simulink model "power_SwitchedReluctanceMotor"  (R2020a)
settings: Solver=FixedStepAuto  StartTime=0.0  StopTime=1  FixedStep=Ts  RelTol=1e-3  AbsTol=1e-5  EnableMultiTasking=on
PreLoadFcn:
  | Ts=1e-6;
  | 
  | % Magnetisation characteristic table of the switched Reluctance Motor:
  | % Table elements =  Flux linkage, in Wb.
  | 
  | FTBL = [
  |     0             0              0             0             0             0
  |     0.3220    0.3050    0.2280    0.1240    0.0220    0.0170
  |     0.3760    0.3570    0.2770    0.1600    0.0420    0.0340
  |     0.3990    0.3850    0.3000    0.1830    0.0640    0.0500
  |     0.4160    0.4020    0.3200    0.2010    0.0840    0.0670
  |     0.4280    0.4150    0.3340    0.2190    0.1030    0.0840
  |     0.4370    0.4260    0.3480    0.2370    0.1230    0.1010
  |     0.4430    0.4330    0.3590    0.2530    0.1420    0.1170
  |     0.4490    0.4390    0.3710    0.2680    0.1610    0.1340
  |     0.4540    0.4440    0.3820    0.2820    0.1790    0.1510
  |     0.4590    0.4490    0.3920    0.2950    0.1970    0.1680
  |     0.4630    0.4530    0.4020    0.3090    0.2140    0.1840
  |     0.4670    0.4570    0.4110    0.3220    0.2310    0.2010
  |     0.4700    0.4620    0.4190    0.3360    0.2460    0.2180
  |     0.4740    0.4650    0.4270    0.3480    0.2610    0.2350
  |     0.4780    0.4690    0.4330    0.3590    0.2770    0.2510
  |     0.4810    0.4730    0.4380    0.3690    0.2910    0.2680
  |     0.4840    0.4770    0.4440    0.3800    0.3050    0.2850
  |     0.4870    0.4790    0.4480    0.3890    0.3200    0.3020];
  | 
  | % Table columns :  Rotor angles, in degrees.
  | 
  | RotorAngles = [
  |     0             10            20            30            40            45];
  | 
  | % Table rows : Stator current, in A.
  | 
  | StatorCurrents = [ 0:size(FTBL,1)-1] * 25;
  | 
  | % In the Switched Reluctance Motor block, select the "plot magnetization curves"
  | % to plot the corresponding characteristic of the above table.
undefined symbols (not defined in the file): DiscIntNeverNeededParam, find_system
libraries: powerlib x40, simulink x3, powerlib_meascontrol x1
settings Model: ExtModeAutoUpdateStatusClock=off  Creator=MathWorks  LastModifiedBy=mahfo
settings SolverCC: AutoScaleAbsTol=off  InsertRTBMode=Auto
settings DataIOCC: LimitDataPoints=on  SaveFormat=Array  SignalLoggingSaveFormat=ModelDataLogs  ReturnWorkspaceOutputs=off  SignalLoggingName=sigsOut
settings OptimizationCC: ExpressionDepthLimit=2147483647  InitFltsAndDblsToZero=on  LifeSpan=inf
settings DebuggingCC: UnderspecifiedInitializationDetection=Classic  MergeDetectMultiDrivingBlocksExec=none  CheckExecutionContextPreStartOutputMsg=on  CheckExecutionContextRuntimeOutputMsg=on  SignalResolutionControl=TryResolveAllWithWarning  MultiTaskDSMMsg=warning  MultiTaskCondExecSysMsg=none  FcnCallInpInsideContextMsg=warning  StateNameClashWarn=warning  SFUnexpectedBacktrackingDiag=warning  SFNoUnconditionalDefaultTransitionDiag=warning  SFExecutionAtInitializationDiag=none  ArithmeticOperatorsInVariantConditions=warning
settings HardwareCC: ProdBitPerPointer=32  ProdBitPerSizeT=32  ProdBitPerPtrDiffT=32  ProdLargestAtomicFloat=None  ProdIntDivRoundTo=Undefined  ProdEndianess=Unspecified  ProdWordSize=32  ProdHWDeviceType=32-bit Generic  TargetUnknown=on
settings ModelReferenceCC: PropagateSignalLabelsOutOfModel=off
settings SFSimCC: SimUseLocalCustomCode=off  CustomCodeUndefinedFunction=UseInterfaceOnly
settings RTWCC: RTWUseLocalCustomCode=off
settings CodeAppCC: StateflowObjectComments=on
settings GRTTargetCC: TargetLangStandard=C89/C90 (ANSI)  CombineOutputUpdateFcns=off  GRTInterface=on
settings ConfigComp: CovMetricSettings=dw  CovHtmlReporting=on  CovSaveCumulativeToWorkspaceVar=on  CovSaveSingleToWorkspaceVar=on  CovExternalEMLEnable=off  CovSFcnEnable=off
settings SimscapeCC: SimscapeNormalizeSystem=off

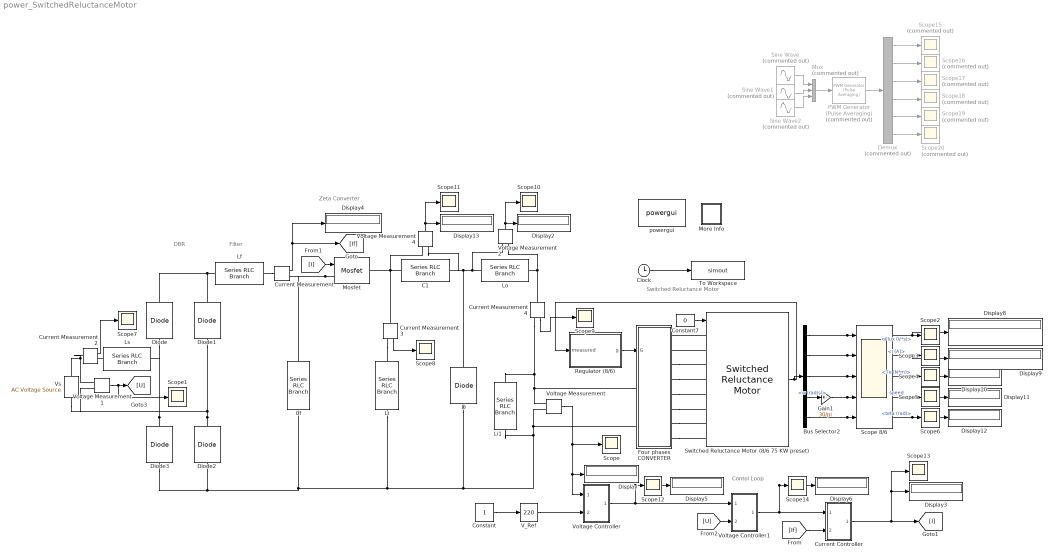
== system power_SwitchedReluctanceMotor ==
  note: Switched Reluctance Motor
  note: Filter
  note: Zeta Converter
  note: DBR
  note: Contol Loop
  Bus Selector2 : BusSelector  OutputSignals=Flux (V*s),I (A),Te (N*m),w (rad/s),teta (rad)
  C1 : powerlib/Elements/Series RLC Branch  LConnTagsString=__new0  RConnTagsString=__new0  BranchType=C  Resistance=1  Inductance=1e-3  SetiL0=off  InitialCurrent=0  Capacitance=1.48e-6  Setx0=off  InitialVoltage=0  Measurements=None
  Cf : powerlib/Elements/Series RLC Branch  LConnTagsString=__new0  RConnTagsString=__new0  BranchType=C  Resistance=1  Inductance=1e-3  SetiL0=off  InitialCurrent=0  Capacitance=1e-6  Setx0=off  InitialVoltage=0  Measurements=None
  Clock : Clock
  Constant : Constant
  Constant7 : Constant  Value=0
  Current Controller : Subsystem
  Current Measurement{,2..4} (4 alike) : powerlib/Measurements/Current Measurement  PhasorSimulation=off  OutputType=Complex  PSBequivalent=0
  D : powerlib/Power Electronics/Diode  Ron=0.001  Lon=0  Vf=0.8  IC=0  UseSnubber=0  Rs=500  Cs=250e-9  Measurements=off
  Demux : Demux  Commented=on  Outputs=6
  Diode{,1..3} (4 alike) : powerlib/Power Electronics/Diode  Ron=0.001  Lon=0  Vf=0.8  IC=0  UseSnubber=0  Rs=500  Cs=250e-9  Measurements=off
  Display{,2..6,8..13} (12 alike) : Display
  Four phases CONVERTER : Subsystem  LoadFcn=find_system(gcs,'FollowLinks', 'on', 'LookUnderMasks', 'all');
  Gain1 : Gain  Gain=30/pi  SaturateOnIntegerOverflow=on  OutDataTypeStr=Inherit: Same as input  ParamDataTypeStr=Inherit: Same as input
  Lf : powerlib/Elements/Series RLC Branch  LConnTagsString=__new0  RConnTagsString=__new0  BranchType=L  Resistance=1  Inductance=1.37e-3  SetiL0=off  InitialCurrent=0  Capacitance=1e-6  Setx0=off  InitialVoltage=0  Measurements=None
  Li : powerlib/Elements/Series RLC Branch  LConnTagsString=__new0  RConnTagsString=__new0  BranchType=L  Resistance=1  Inductance=1e-3  SetiL0=off  InitialCurrent=0  Capacitance=1e-6  Setx0=off  InitialVoltage=0  Measurements=None
  Li1 : powerlib/Elements/Series RLC Branch  LConnTagsString=__new0  RConnTagsString=__new0  BranchType=C  Resistance=10  Inductance=100  SetiL0=off  InitialCurrent=0  Capacitance=1500e-6  Setx0=off  InitialVoltage=0  Measurements=None
  Lo : powerlib/Elements/Series RLC Branch  LConnTagsString=__new0  RConnTagsString=__new0  BranchType=L  Resistance=1  Inductance=4.51e-3  SetiL0=off  InitialCurrent=0  Capacitance=1e-6  Setx0=off  InitialVoltage=0  Measurements=None
  Ls : powerlib/Elements/Series RLC Branch  LConnTagsString=__new0  RConnTagsString=__new0  BranchType=L  Resistance=1  Inductance=4.38e-3  SetiL0=off  InitialCurrent=0  Capacitance=1e-6  Setx0=off  InitialVoltage=0  Measurements=None
  More Info : Subsystem
      settings: OpenFcn=showdemo(bdroot(gcb))
      mask Display: disp('?')
  Mosfet : powerlib/Power Electronics/Mosfet  Ron=0.1  Lon=0  Rd=0.01  Vfd=0  IC=0  Rs=1e5  Cs=inf  Measurements=off
  Mux : Mux  Commented=on  Inputs=3
  PWM Generator (Pulse Averaging) : powerlib_meascontrol/Pulse & Signal Generators/PWM Generator (Pulse Averaging)  Commented=on  GeneratorType=Two-level, three-phase  Fc=2000  InitialPhase=0  Ts=Ts
      settings: SourceProductBaseCode=PS
  Regulator (8/6) : Subsystem  mask{Iref=50, initpos=[0,-15,-30,-45], TurnOn=37.5, TurnOff=52.5}
      mask prompts: Iref "Reference current"; initpos "initial positions"; TurnOn "Turn-on angle (deg)"; TurnOff "Turn-off angle (deg)"
  Scope{,1..14} (15 alike) : Scope
  Scope 8/6 : Scope  NumInputPorts=5
  Scope{15..20} (6 alike) : Scope  Commented=on
  Sine Wave : Sin  Commented=on  SampleTime=0
  Sine Wave1 : Sin  Commented=on  SampleTime=0
  Sine Wave2 : Sin  Commented=on  SampleTime=0
  Switched Reluctance Motor (8/6 75 KW preset) : powerlib/Machines/Switched Reluctance Motor  MachineType="8/6  (75 kw preset model)"  StatorResistance=0.05  Inertia=0.01  Friction=0.005  InitialSpeed=[0,0]  TsPowergui=0  TsBlock=Ts  MachineModel=Specific model  Lq=0.67e-3  Ld=23.6e-3  Lsat=0.15e-3  MaximumCurrent=450  MaximumFluxLinkage=0.486  Source=Dialog  MagnetisationCharacteristic=FTBL  RotorAngleVector=RotorAngles  StatorCurrentVector=StatorCurrents  PlotCurves=off
      settings: SourceProductBaseCode=MT,PS
  To Workspace : ToWorkspace  VariableName=simout  SaveFormat=Timeseries  SampleTime=-1
  V_Ref : simulink/Math Operations/Slider Gain  gain=220  low=0  high=440
  Voltage Controller : Subsystem
  Voltage Controller1 : Subsystem
  Voltage Measurement{,1..2,4} (4 alike) : powerlib/Measurements/Voltage Measurement  PhasorSimulation=off  OutputType=Complex  PSBequivalent=0
  Vs : powerlib/Electrical Sources/AC Voltage Source  Amplitude=320  Phase=0  Frequency=200  SampleTime=0  Measurements=None  BusType=swing  Pref=10e3  Qref=0  Qmin=-inf  Qmax=+inf
  powergui : powerlib/powergui  Priority=2  SimulationMode=Discrete  SampleTime=Ts  frequency=60  Iterations=50  frequencyindice=0  Pbase=100e6  ErrMax=1e-4  UnitsV=kV  UnitsW=MW  buscounter=0  FunctionMessages=off  echomessages=off  EnableUseOfTLC=off  CurrentSourceSwitches=off  DisableSnubberDevices=off  DisableRonSwitches=off  DisableVfSwitches=off  DisplayEquations=off  AutomaticDiscreteSolvers=off  SolverType=Tustin/Backward Euler (TBE)  Interpol=off  ExternalGateDelay=off  methode=off  Ts=0  x0status=blocks  SPID=off  SwTol=0  HookPort=off  NonlinearTolerance=0  nMaxIteration=15  ContinueOnMaxIteration=off  RestoreLinks=warning  ResistiveCurrentMeasurement=off  Frange=[0:2:500]  Ylog=off  Xlog=on  ShowGrid=off  save=off  variable=ZData  structure=0  ZoomFFT=on  StartTime=0.0  cycles=1  DisplayStyle=1  fundamental=60  FreqAxis=off  MaxFrequency=1000  frequencyindicesteady=1  RmsSteady=1  display=off
  wires:
  Constant7/1 -> Switched Reluctance Motor (8/6 75 KW preset)/1
  Switched Reluctance Motor (8/6 75 KW preset)/1 -> Bus Selector2/1, Regulator (8/6)/1(measured)
  Regulator (8/6)/1(g) -> Four phases CONVERTER/1(G)
  Bus Selector2/1 -> Display8/1, Scope2/1, Scope 8/6/1  "<Flux (V*s)>"
  Bus Selector2/2 -> Scope 8/6/2, Display9/1, Scope3/1  "<I (A)>"
  Bus Selector2/3 -> Display10/1, Scope4/1, Scope 8/6/3  "<Te (N*m)>"
  Bus Selector2/4 -> Gain1/1  "<w (rad/s)>"
  Gain1/1 -> Display11/1, Scope5/1, Scope 8/6/4  "speed"
  ? -> ?
  Voltage Measurement/1 -> Voltage Controller/1(In1), Display/1, Scope/1
  Bus Selector2/5 -> Scope 8/6/5, Display12/1, Scope6/1  "<teta (rad)>"
  Current Measurement/1 -> Display4/1, [If]
  [If] -> Current Controller/2(In2)
  Current Controller/1(Out1) -> Display3/1, Scope13/1, [I]
  Clock/1 -> To Workspace/1
  Constant/1 -> V_Ref/1
  V_Ref/1 -> Voltage Controller/2(In2)
  Voltage Measurement1/1 -> Scope1/1, [U]
  Voltage Controller/1(Out1) -> Voltage Controller1/1(In1), Display5/1, Scope12/1
  [U] -> Voltage Controller1/2(In2)
  Current Measurement2/1 -> Scope7/1
  Current Measurement3/1 -> Scope8/1
  Current Measurement4/1 -> Scope9/1
  Voltage Measurement2/1 -> Scope10/1, Display2/1
  Voltage Measurement4/1 -> Display13/1, Scope11/1
  PWM Generator (Pulse Averaging)/1 -> Demux/1
  Sine Wave/1 -> Mux/1
  Sine Wave1/1 -> Mux/2
  Sine Wave2/1 -> Mux/3
  Mux/1 -> PWM Generator (Pulse Averaging)/1
  Demux/1 -> Scope15/1
  Demux/2 -> Scope16/1
  Demux/3 -> Scope17/1
  Demux/4 -> Scope18/1
  Demux/5 -> Scope19/1
  Demux/6 -> Scope20/1
  Voltage Controller1/1(Out1) -> Current Controller/1(In1), Display6/1, Scope14/1
  [I] -> Mosfet/1
  connections:
  Switched Reluctance Motor (8/6 75 KW preset)/LConn2 -- Four phases CONVERTER/RConn2
  Four phases CONVERTER/RConn3 -- Switched Reluctance Motor (8/6 75 KW preset)/LConn3
  Switched Reluctance Motor (8/6 75 KW preset)/LConn1 -- Four phases CONVERTER/RConn1
  Four phases CONVERTER/RConn4 -- Switched Reluctance Motor (8/6 75 KW preset)/LConn4
  Four phases CONVERTER/RConn5 -- Switched Reluctance Motor (8/6 75 KW preset)/LConn5
  Four phases CONVERTER/RConn6 -- Switched Reluctance Motor (8/6 75 KW preset)/LConn6
  Four phases CONVERTER/RConn7 -- Switched Reluctance Motor (8/6 75 KW preset)/LConn7
  Four phases CONVERTER/RConn8 -- Switched Reluctance Motor (8/6 75 KW preset)/LConn8
  Current Measurement4/LConn1 -- Voltage Measurement2/LConn2 -- Lo/RConn1
  Mosfet/LConn1 -- Current Measurement/RConn1 -- Cf/LConn1
  C1/LConn1 -- Voltage Measurement4/LConn2 -- Current Measurement3/LConn1 -- Mosfet/RConn1
  Diode2/RConn1 -- Vs/LConn1 -- Voltage Measurement1/LConn2 -- Diode1/LConn1
  Lo/LConn1 -- Voltage Measurement4/LConn1 -- C1/RConn1 -- D/RConn1 -- Voltage Measurement2/LConn1
  Diode/RConn1 -- Lf/LConn1 -- Diode1/RConn1
  Diode3/RConn1 -- Diode/LConn1 -- Ls/RConn1
  Voltage Measurement1/LConn1 -- Current Measurement2/LConn1 -- Vs/RConn1
  Voltage Measurement/LConn2 -- Four phases CONVERTER/LConn2 -- Li1/LConn1 -- D/LConn1 -- Li/LConn1 -- Diode3/LConn1 -- Diode2/LConn1 -- Cf/RConn1
  Current Measurement2/RConn1 -- Ls/LConn1
  Current Measurement4/RConn1 -- Voltage Measurement/LConn1 -- Four phases CONVERTER/LConn1 -- Li1/RConn1
  Current Measurement3/RConn1 -- Li/RConn1
  Lf/RConn1 -- Current Measurement/LConn1

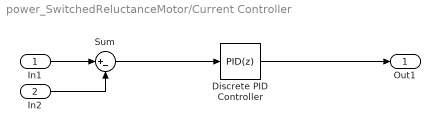
== system power_SwitchedReluctanceMotor/Current Controller ==
  In1 : Inport
  In2 : Inport  Port=2
  Discrete PID Controller : simulink/Continuous/PID Controller  Controller=PID  Form=Parallel  TimeDomain=Discrete-time  UseExternalTs=off  SampleTime=-1  IntegratorMethod=Forward Euler  FilterMethod=Forward Euler  ControllerParametersSource=internal  P=1  I=1  D=0  UseFilter=on  N=100  TunerSelectOption=Transfer Function Based (PID Tuner App)  InitialConditionSource=internal  InitialConditionForIntegrator=0  InitialConditionForFilter=0  DifferentiatorICPrevScaledInput=0  ExternalReset=none  TrackingMode=off  Kt=1  LimitOutput=off  UpperSaturationLimit=inf  LowerSaturationLimit=-inf  LinearizeAsGain=off  AntiWindupMode=none  Kb=1  POutMin=[]  POutMax=[]  IOutMin=[]  IOutMax=[]  DOutMin=[]  DOutMax=[]  NOutMin=[]  NOutMax=[]  SumOutMin=[]  SumOutMax=[]  SaturationOutMin=[]  SaturationOutMax=[]  PParamMin=[]  PParamMax=[]  IParamMin=[]  IParamMax=[]  DParamMin=[]  DParamMax=[]  NParamMin=[]  NParamMax=[]  KbParamMin=[]  KbParamMax=[]  KtParamMin=[]  KtParamMax=[]  KbOutMin=[]  KbOutMax=[]  KtOutMin=[]  KtOutMax=[]  IntegratorOutMin=[]  IntegratorOutMax=[]  FilterOutMin=[]  FilterOutMax=[]  SumI1OutMin=[]  SumI1OutMax=[]  SumI2OutMin=[]  SumI2OutMax=[]  SumI3OutMin=[]  SumI3OutMax=[]  SumI4OutMin=[]  SumI4OutMax=[]  SumDOutMin=[]  SumDOutMax=[]  DifferentiatorOutMin=[]  DifferentiatorOutMax=[]  FilterDiffOutCoefMin=[]  FilterDiffOutCoefMax=[]  ReciprocalOutMin=[]  ReciprocalOutMax=[]  SumDenOutMin=[]  SumDenOutMax=[]  SumNumOutMin=[]  SumNumOutMax=[]  DivideOutMin=[]  DivideOutMax=[]  UdiffTsProdOutMin=[]  UdiffTsProdOutMax=[]  NTsProdOutMin=[]  NTsProdOutMax=[]  UintegralTsProdOutMin=[]  UintegralTsProdOutMax=[]  UngainTsProdOutMin=[]  UngainTsProdOutMax=[]  IntegratorContinuousStateAttributes=''  IntegratorStateMustResolveToSignalObject=off  IntegratorRTWStateStorageClass=Auto  FilterContinuousStateAttributes=''  FilterStateMustResolveToSignalObject=off  FilterRTWStateStorageClass=Auto  ParallelPVariant=InternalParameters  IdealPVariant=Disabled  IVariant=InternalParameters  DVariant=InternalParameters  IntegratorVariant=Discrete  SatVariant=Disabled  AWVariant=Passthrough  PCopyVariant=Disabled  TRVariant=Disabled  FdbkBlocksVariant=Forward  IdealPFdbkVariant=Disabled  SatFdbkVariant=Disabled  DerivativeFilterVariant=ForwardEulerFilter  NVariant=InternalParameters  NCopyVariant=Disabled  FilterICVariant=InternalICsFilter  IntegratorICVariant=InternalICs  ExternalResetVariant=Disabled  TRSumVariant=Passthrough  SumFdbkVariant=Disabled  SumVariant=Sum_PID  TsampFilterVariant=InternalTs  TsampNgainVariant=Passthrough  TsampIntegralVariant=Passthrough
  Sum : Sum  Inputs=|+-
  Out1 : Outport
  wires:
  Sum/1 -> Discrete PID Controller/1
  In1/1 -> Sum/1
  In2/1 -> Sum/2
  Discrete PID Controller/1 -> Out1/1

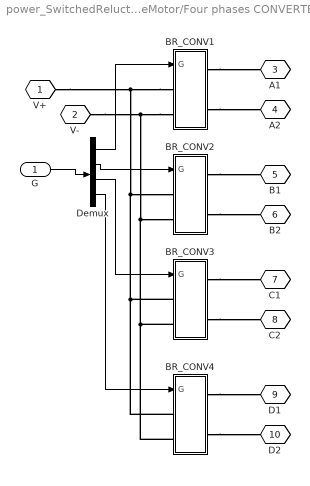
== system power_SwitchedReluctanceMotor/Four phases CONVERTER ==
  G : Inport
  BR_CONV1 : Subsystem
  BR_CONV2 : Subsystem
  BR_CONV3 : Subsystem
  BR_CONV4 : Subsystem
  Demux : Demux
      settings: DisplayOption=none
  V+ : PMIOPort  Tag=PMCPort  Side=Left
  V- : PMIOPort  Tag=PMCPort  Port=2  Side=Left
  A1 : PMIOPort  Tag=PMCPort  Port=3  Side=Right
  A2 : PMIOPort  Tag=PMCPort  Port=4  Side=Right
  B1 : PMIOPort  Tag=PMCPort  Port=5  Side=Right
  B2 : PMIOPort  Tag=PMCPort  Port=6  Side=Right
  C1 : PMIOPort  Tag=PMCPort  Port=7  Side=Right
  C2 : PMIOPort  Tag=PMCPort  Port=8  Side=Right
  D1 : PMIOPort  Tag=PMCPort  Port=9  Side=Right
  D2 : PMIOPort  Tag=PMCPort  Port=10  Side=Right
  wires:
  Demux/4 -> BR_CONV4/1(G)
  Demux/3 -> BR_CONV3/1(G)
  Demux/1 -> BR_CONV1/1(G)
  Demux/2 -> BR_CONV2/1(G)
  G/1 -> Demux/1
  connections:
  BR_CONV4/RConn1 -- D1/RConn1
  BR_CONV4/RConn2 -- D2/RConn1
  BR_CONV3/RConn2 -- C2/RConn1
  BR_CONV3/RConn1 -- C1/RConn1
  BR_CONV2/RConn2 -- B2/RConn1
  BR_CONV2/RConn1 -- B1/RConn1
  BR_CONV1/RConn2 -- A2/RConn1
  BR_CONV1/RConn1 -- A1/RConn1
  BR_CONV1/LConn2 -- V-/RConn1 -- BR_CONV3/LConn2 -- BR_CONV4/LConn2 -- BR_CONV2/LConn2
  BR_CONV1/LConn1 -- V+/RConn1 -- BR_CONV3/LConn1 -- BR_CONV4/LConn1 -- BR_CONV2/LConn1

== system power_SwitchedReluctanceMotor/More Info ==

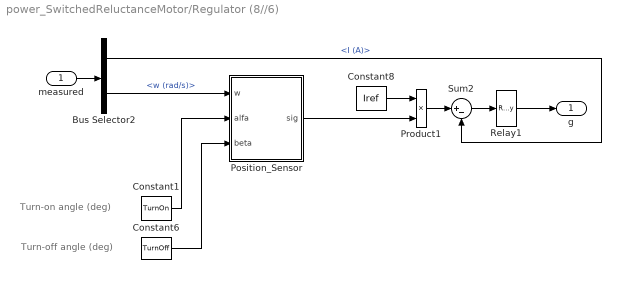
== system power_SwitchedReluctanceMotor/Regulator (8//6) ==
  note: Turn-on angle (deg)
  note: Turn-off angle (deg)
  measured : Inport
  Bus Selector2 : BusSelector  OutputSignals=I (A),w (rad/s)
  Constant1 : Constant  Value=TurnOn
  Constant6 : Constant  Value=TurnOff
  Constant8 : Constant  Value=Iref
  Position_Sensor : Subsystem
  Product1 : Product  SaturateOnIntegerOverflow=on  OutDataTypeStr=Inherit: Same as first input
  Relay1 : Relay  OnSwitchValue=5  OffSwitchValue=-5  SampleTime=Ts
  Sum2 : Sum  Inputs=|+-  SaturateOnIntegerOverflow=on
  g : Outport  VectorParamsAs1DForOutWhenUnconnected=off
  wires:
  Bus Selector2/2 -> Position_Sensor/1(w)  "<w (rad/s)>"
  Bus Selector2/1 -> Sum2/2  "<I (A)>"
  measured/1 -> Bus Selector2/1
  Relay1/1 -> g/1
  Position_Sensor/1(sig) -> Product1/2
  Constant8/1 -> Product1/1
  Product1/1 -> Sum2/1
  Sum2/1 -> Relay1/1
  Constant6/1 -> Position_Sensor/3(beta)
  Constant1/1 -> Position_Sensor/2(alfa)

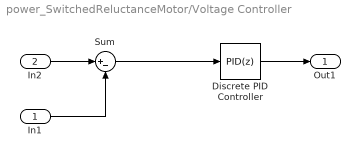
== system power_SwitchedReluctanceMotor/Voltage Controller ==
  In1 : Inport
  In2 : Inport  Port=2
  Discrete PID Controller : simulink/Continuous/PID Controller  Controller=PID  Form=Parallel  TimeDomain=Discrete-time  UseExternalTs=off  SampleTime=-1  IntegratorMethod=Forward Euler  FilterMethod=Forward Euler  ControllerParametersSource=internal  P=1  I=1  D=0  UseFilter=on  N=100  TunerSelectOption=Transfer Function Based (PID Tuner App)  InitialConditionSource=internal  InitialConditionForIntegrator=0  InitialConditionForFilter=0  DifferentiatorICPrevScaledInput=0  ExternalReset=none  TrackingMode=off  Kt=1  LimitOutput=off  UpperSaturationLimit=inf  LowerSaturationLimit=-inf  LinearizeAsGain=off  AntiWindupMode=none  Kb=1  POutMin=[]  POutMax=[]  IOutMin=[]  IOutMax=[]  DOutMin=[]  DOutMax=[]  NOutMin=[]  NOutMax=[]  SumOutMin=[]  SumOutMax=[]  SaturationOutMin=[]  SaturationOutMax=[]  PParamMin=[]  PParamMax=[]  IParamMin=[]  IParamMax=[]  DParamMin=[]  DParamMax=[]  NParamMin=[]  NParamMax=[]  KbParamMin=[]  KbParamMax=[]  KtParamMin=[]  KtParamMax=[]  KbOutMin=[]  KbOutMax=[]  KtOutMin=[]  KtOutMax=[]  IntegratorOutMin=[]  IntegratorOutMax=[]  FilterOutMin=[]  FilterOutMax=[]  SumI1OutMin=[]  SumI1OutMax=[]  SumI2OutMin=[]  SumI2OutMax=[]  SumI3OutMin=[]  SumI3OutMax=[]  SumI4OutMin=[]  SumI4OutMax=[]  SumDOutMin=[]  SumDOutMax=[]  DifferentiatorOutMin=[]  DifferentiatorOutMax=[]  FilterDiffOutCoefMin=[]  FilterDiffOutCoefMax=[]  ReciprocalOutMin=[]  ReciprocalOutMax=[]  SumDenOutMin=[]  SumDenOutMax=[]  SumNumOutMin=[]  SumNumOutMax=[]  DivideOutMin=[]  DivideOutMax=[]  UdiffTsProdOutMin=[]  UdiffTsProdOutMax=[]  NTsProdOutMin=[]  NTsProdOutMax=[]  UintegralTsProdOutMin=[]  UintegralTsProdOutMax=[]  UngainTsProdOutMin=[]  UngainTsProdOutMax=[]  IntegratorContinuousStateAttributes=''  IntegratorStateMustResolveToSignalObject=off  IntegratorRTWStateStorageClass=Auto  FilterContinuousStateAttributes=''  FilterStateMustResolveToSignalObject=off  FilterRTWStateStorageClass=Auto  ParallelPVariant=InternalParameters  IdealPVariant=Disabled  IVariant=InternalParameters  DVariant=InternalParameters  IntegratorVariant=Discrete  SatVariant=Disabled  AWVariant=Passthrough  PCopyVariant=Disabled  TRVariant=Disabled  FdbkBlocksVariant=Forward  IdealPFdbkVariant=Disabled  SatFdbkVariant=Disabled  DerivativeFilterVariant=ForwardEulerFilter  NVariant=InternalParameters  NCopyVariant=Disabled  FilterICVariant=InternalICsFilter  IntegratorICVariant=InternalICs  ExternalResetVariant=Disabled  TRSumVariant=Passthrough  SumFdbkVariant=Disabled  SumVariant=Sum_PID  TsampFilterVariant=InternalTs  TsampNgainVariant=Passthrough  TsampIntegralVariant=Passthrough
  Sum : Sum  Inputs=|+-
  Out1 : Outport
  wires:
  In2/1 -> Sum/1
  In1/1 -> Sum/2
  Sum/1 -> Discrete PID Controller/1
  Discrete PID Controller/1 -> Out1/1

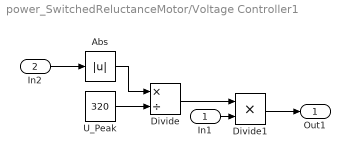
== system power_SwitchedReluctanceMotor/Voltage Controller1 ==
  In1 : Inport
  In2 : Inport  Port=2
  Abs : Abs
  Divide : Product  Inputs=*/
  Divide1 : Product  Inputs=**
  U_Peak : Constant  Value=320
  Out1 : Outport
  wires:
  In2/1 -> Abs/1
  U_Peak/1 -> Divide/2
  Divide/1 -> Divide1/1
  In1/1 -> Divide1/2
  Divide1/1 -> Out1/1
  Abs/1 -> Divide/1

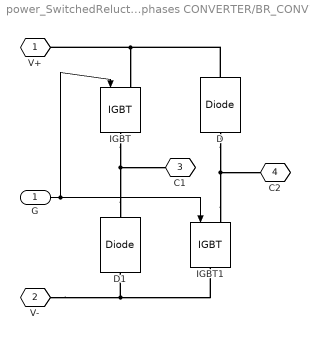
== system power_SwitchedReluctanceMotor/Four phases CONVERTER/BR_CONV1 ==
  G : Inport
  D : powerlib/Power Electronics/Diode  Ron=1e-3  Lon=0  Vf=0.8  IC=0  UseSnubber=off  Rs=1000  Cs=inf  Measurements=off
      settings: SourceProductBaseCode=MT,PS
  D1 : powerlib/Power Electronics/Diode  Ron=1e-3  Lon=0  Vf=0.8  IC=0  UseSnubber=off  Rs=1000  Cs=inf  Measurements=off
      settings: SourceProductBaseCode=MT,PS
  IGBT : powerlib/Power Electronics/IGBT  Ron=1e-3  Lon=0  Vf=1  Tf=0  Tt=0  IC=0  Rs=200  Cs=0.1e-6  Measurements=off
      settings: SourceProductBaseCode=MT,PS
  IGBT1 : powerlib/Power Electronics/IGBT  Ron=1e-3  Lon=0  Vf=1  Tf=0  Tt=0  IC=0  Rs=200  Cs=0.1e-6  Measurements=off
      settings: SourceProductBaseCode=MT,PS
  V+ : PMIOPort  Tag=PMCPort  Side=Left
  V- : PMIOPort  Tag=PMCPort  Port=2  Side=Left
  C1 : PMIOPort  Tag=PMCPort  Port=3  Side=Right
  C2 : PMIOPort  Tag=PMCPort  Port=4  Side=Right
  wires:
  G/1 -> IGBT/1, IGBT1/1
  connections:
  D1/LConn1 -- V-/RConn1 -- IGBT1/RConn1
  IGBT1/LConn1 -- D/LConn1 -- C2/RConn1
  D1/RConn1 -- IGBT/RConn1 -- C1/RConn1
  D/RConn1 -- V+/RConn1 -- IGBT/LConn1

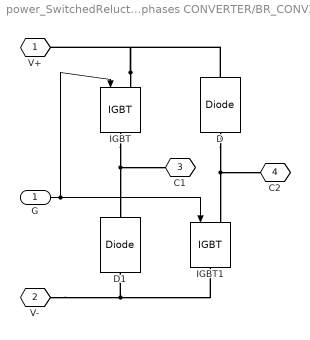
== system power_SwitchedReluctanceMotor/Four phases CONVERTER/BR_CONV2 ==
  G : Inport
  D : powerlib/Power Electronics/Diode  Ron=1e-3  Lon=0  Vf=0.8  IC=0  UseSnubber=off  Rs=1000  Cs=inf  Measurements=off
      settings: SourceProductBaseCode=MT,PS
  D1 : powerlib/Power Electronics/Diode  Ron=1e-3  Lon=0  Vf=0.8  IC=0  UseSnubber=off  Rs=1000  Cs=inf  Measurements=off
      settings: SourceProductBaseCode=MT,PS
  IGBT : powerlib/Power Electronics/IGBT  Ron=1e-3  Lon=0  Vf=1  Tf=0  Tt=0  IC=0  Rs=200  Cs=0.1e-6  Measurements=off
      settings: SourceProductBaseCode=MT,PS
  IGBT1 : powerlib/Power Electronics/IGBT  Ron=1e-3  Lon=0  Vf=1  Tf=0  Tt=0  IC=0  Rs=200  Cs=0.1e-6  Measurements=off
      settings: SourceProductBaseCode=MT,PS
  V+ : PMIOPort  Tag=PMCPort  Side=Left
  V- : PMIOPort  Tag=PMCPort  Port=2  Side=Left
  C1 : PMIOPort  Tag=PMCPort  Port=3  Side=Right
  C2 : PMIOPort  Tag=PMCPort  Port=4  Side=Right
  wires:
  G/1 -> IGBT1/1, IGBT/1
  connections:
  IGBT/LConn1 -- V+/RConn1 -- D/RConn1
  IGBT/RConn1 -- D1/RConn1 -- C1/RConn1
  D/LConn1 -- IGBT1/LConn1 -- C2/RConn1
  V-/RConn1 -- D1/LConn1 -- IGBT1/RConn1

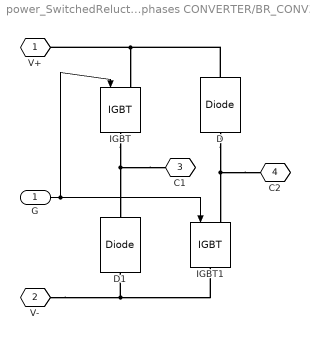
== system power_SwitchedReluctanceMotor/Four phases CONVERTER/BR_CONV3 ==
  G : Inport
  D : powerlib/Power Electronics/Diode  Ron=1e-3  Lon=0  Vf=0.8  IC=0  UseSnubber=off  Rs=1000  Cs=inf  Measurements=off
      settings: SourceProductBaseCode=MT,PS
  D1 : powerlib/Power Electronics/Diode  Ron=1e-3  Lon=0  Vf=0.8  IC=0  UseSnubber=off  Rs=1000  Cs=inf  Measurements=off
      settings: SourceProductBaseCode=MT,PS
  IGBT : powerlib/Power Electronics/IGBT  Ron=1e-3  Lon=0  Vf=1  Tf=0  Tt=0  IC=0  Rs=200  Cs=0.1e-6  Measurements=off
      settings: SourceProductBaseCode=MT,PS
  IGBT1 : powerlib/Power Electronics/IGBT  Ron=1e-3  Lon=0  Vf=1  Tf=0  Tt=0  IC=0  Rs=200  Cs=0.1e-6  Measurements=off
      settings: SourceProductBaseCode=MT,PS
  V+ : PMIOPort  Tag=PMCPort  Side=Left
  V- : PMIOPort  Tag=PMCPort  Port=2  Side=Left
  C1 : PMIOPort  Tag=PMCPort  Port=3  Side=Right
  C2 : PMIOPort  Tag=PMCPort  Port=4  Side=Right
  wires:
  G/1 -> IGBT/1, IGBT1/1
  connections:
  IGBT1/RConn1 -- D1/LConn1 -- V-/RConn1
  C2/RConn1 -- IGBT1/LConn1 -- D/LConn1
  C1/RConn1 -- D1/RConn1 -- IGBT/RConn1
  D/RConn1 -- V+/RConn1 -- IGBT/LConn1

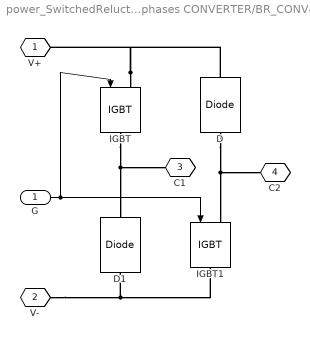
== system power_SwitchedReluctanceMotor/Four phases CONVERTER/BR_CONV4 ==
  G : Inport
  D : powerlib/Power Electronics/Diode  Ron=1e-3  Lon=0  Vf=0.8  IC=0  UseSnubber=off  Rs=1000  Cs=inf  Measurements=off
      settings: SourceProductBaseCode=MT,PS
  D1 : powerlib/Power Electronics/Diode  Ron=1e-3  Lon=0  Vf=0.8  IC=0  UseSnubber=off  Rs=1000  Cs=inf  Measurements=off
      settings: SourceProductBaseCode=MT,PS
  IGBT : powerlib/Power Electronics/IGBT  Ron=1e-3  Lon=0  Vf=1  Tf=0  Tt=0  IC=0  Rs=200  Cs=0.1e-6  Measurements=off
      settings: SourceProductBaseCode=MT,PS
  IGBT1 : powerlib/Power Electronics/IGBT  Ron=1e-3  Lon=0  Vf=1  Tf=0  Tt=0  IC=0  Rs=200  Cs=0.1e-6  Measurements=off
      settings: SourceProductBaseCode=MT,PS
  V+ : PMIOPort  Tag=PMCPort  Side=Left
  V- : PMIOPort  Tag=PMCPort  Port=2  Side=Left
  C1 : PMIOPort  Tag=PMCPort  Port=3  Side=Right
  C2 : PMIOPort  Tag=PMCPort  Port=4  Side=Right
  wires:
  G/1 -> IGBT1/1, IGBT/1
  connections:
  IGBT/LConn1 -- V+/RConn1 -- D/RConn1
  IGBT/RConn1 -- D1/RConn1 -- C1/RConn1
  D/LConn1 -- IGBT1/LConn1 -- C2/RConn1
  V-/RConn1 -- D1/LConn1 -- IGBT1/RConn1

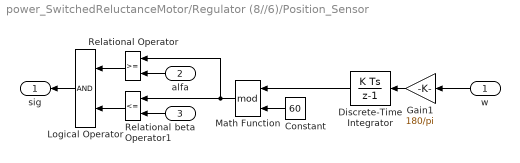
== system power_SwitchedReluctanceMotor/Regulator (8//6)/Position_Sensor ==
  w : Inport
  alfa : Inport  Port=2
  beta : Inport  Port=3
  Constant : Constant  Value=60
  Discrete-Time Integrator : DiscreteIntegrator  InitialCondition=initpos  SampleTime=Ts  ICPrevOutput=DiscIntNeverNeededParam  ICPrevScaledInput=DiscIntNeverNeededParam
  Gain1 : Gain  Gain=180/pi  SaturateOnIntegerOverflow=on  OutDataTypeStr=Inherit: Same as input  ParamDataTypeStr=Inherit: Same as input
  Logical Operator : Logic  AllPortsSameDT=off
  Math Function : Math  Operator=mod  SignedPower=on  SaturateOnIntegerOverflow=on
  Relational Operator : RelationalOperator  RndMeth=Nearest
  Relational Operator1 : RelationalOperator  Operator=<=  RndMeth=Nearest
  sig : Outport  VectorParamsAs1DForOutWhenUnconnected=off
  wires:
  Logical Operator/1 -> sig/1
  w/1 -> Gain1/1
  Math Function/1 -> Relational Operator/1, Relational Operator1/1
  Relational Operator1/1 -> Logical Operator/2
  Gain1/1 -> Discrete-Time Integrator/1
  beta/1 -> Relational Operator1/2
  alfa/1 -> Relational Operator/2
  Relational Operator/1 -> Logical Operator/1
  Constant/1 -> Math Function/2
  Discrete-Time Integrator/1 -> Math Function/1
